simulink subsystem "aTaskGrad"  (R2023a)
settings: Solver=VariableStepAuto  StartTime=0.0  StopTime=10.0  RelTol=1e-3
settings Model: Creator=KozlovM  LastModifiedBy=motya

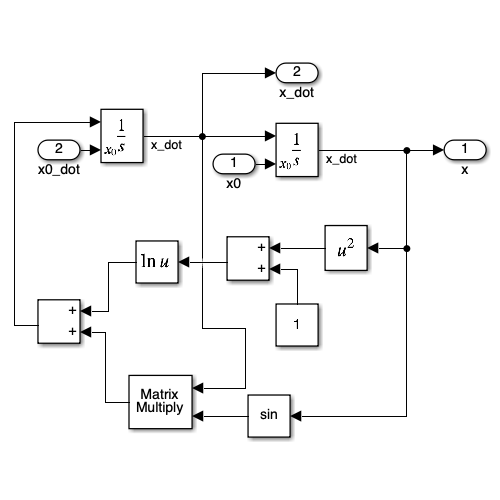
[thumbnail: Simulink's stored preview of the top-level diagram]
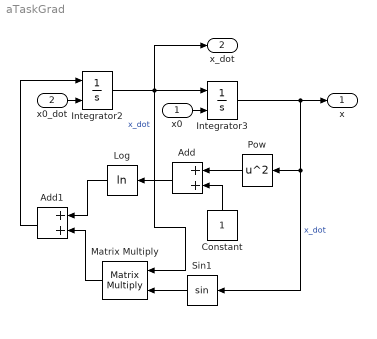
== system aTaskGrad ==
  x0 : Inport
  x0_dot : Inport  Port=2
  Add : Sum
  Add1 : Sum
  Constant : Constant
  Integrator2 : Integrator  InitialConditionSource=external
  Integrator3 : Integrator  InitialConditionSource=external
  Log : Math  Operator=log
  Matrix Multiply : Product  Multiplication=Matrix(*)
  Pow : Math  Operator=square  RndMeth=Zero
  Sin1 : Trigonometry
  x : Outport
  x_dot : Outport  Port=2
  wires:
  Constant/1 -> Add/2
  Add/1 -> Log/1
  Pow/1 -> Add/1
  Sin1/1 -> Matrix Multiply/2
  Log/1 -> Add1/1
  Matrix Multiply/1 -> Add1/2
  x0_dot/1 -> Integrator2/2
  Add1/1 -> Integrator2/1
  Integrator2/1 -> x_dot/1, Matrix Multiply/1, Integrator3/1  "x_dot"
  x0/1 -> Integrator3/2
  Integrator3/1 -> Sin1/1, Pow/1, x/1  "x_dot"
